simulink model "task_1"  (R2023b)
settings: Solver=FixedStepAuto  StartTime=0.0  StopTime=10  FixedStep=1e-3  RelTol=1e-3
values from neighbouring files (symbols this model uses):
  lambda = 4    [task_1.m]
  theta = 6    [task_1.m]
  x_init = 8    [task_1.m]
  x_m_init = 7    [task_1.m]
settings Model: Creator=nguye  LastModifiedBy=nguye

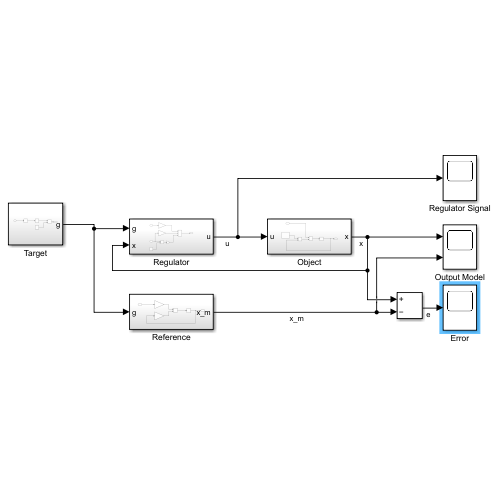
[thumbnail: Simulink's stored preview of the top-level diagram]
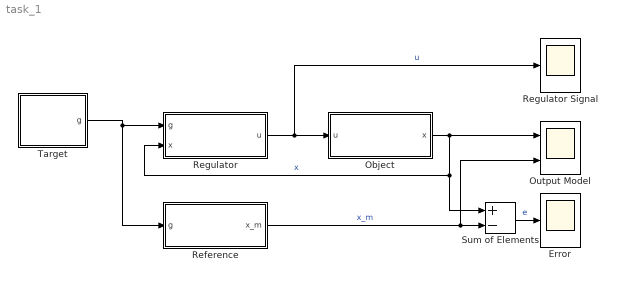
== system task_1 ==
  Error : Scope
  Object : Subsystem
  Output Model : Scope  NumInputPorts=2
  Reference : Subsystem
  Regulator : Subsystem
  Regulator Signal : Scope
  Sum of Elements : Sum  Inputs=+-
  Target : Subsystem
  wires:
  Target/1(g) -> Reference/1(g), Regulator/1(g)
  Regulator/1(u) -> Regulator Signal/1, Object/1(u)  "u"
  Object/1(x) -> Output Model/1, Sum of Elements/1, Regulator/2(x)  "x"
  Reference/1(x_m) -> Output Model/2, Sum of Elements/2  "x_m"
  Sum of Elements/1 -> Error/1  "e"

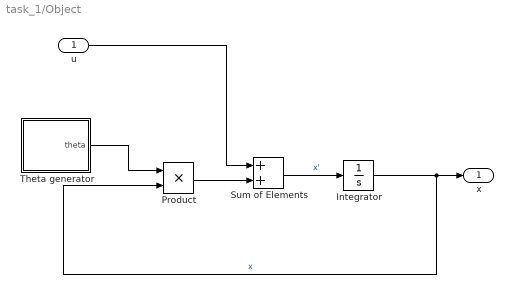
== system task_1/Object ==
  u : Inport
  Integrator : Integrator  InitialCondition=x_init
  Product : Product
  Sum of Elements : Sum
  Theta generator : Subsystem
  x : Outport
  wires:
  Integrator/1 -> Product/2, x/1  "x"
  Product/1 -> Sum of Elements/2
  Sum of Elements/1 -> Integrator/1  "x'"
  u/1 -> Sum of Elements/1
  Theta generator/1(theta) -> Product/1

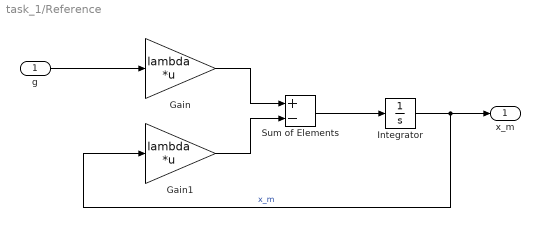
== system task_1/Reference ==
  g : Inport
  Gain : Gain  Gain=lambda  Multiplication=Matrix(K*u)
  Gain1 : Gain  Gain=lambda  Multiplication=Matrix(K*u)
  Integrator : Integrator  InitialCondition=x_m_init
  Sum of Elements : Sum  Inputs=+-
  x_m : Outport
  wires:
  Sum of Elements/1 -> Integrator/1
  Integrator/1 -> Gain1/1, x_m/1  "x_m"
  Gain/1 -> Sum of Elements/1
  g/1 -> Gain/1
  Gain1/1 -> Sum of Elements/2

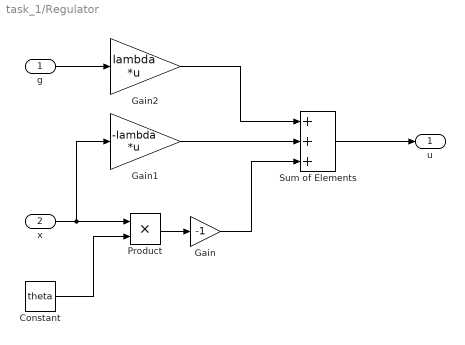
== system task_1/Regulator ==
  g : Inport
  x : Inport  Port=2
  Constant : Constant  Value=theta
  Gain : Gain  Gain=-1
  Gain1 : Gain  Gain=-lambda  Multiplication=Matrix(K*u)
  Gain2 : Gain  Gain=lambda  Multiplication=Matrix(K*u)
  Product : Product
  Sum of Elements : Sum  Inputs=+++
  u : Outport
  wires:
  x/1 -> Product/1, Gain1/1
  g/1 -> Gain2/1
  Sum of Elements/1 -> u/1
  Gain2/1 -> Sum of Elements/1
  Gain1/1 -> Sum of Elements/2
  Product/1 -> Gain/1
  Constant/1 -> Product/2
  Gain/1 -> Sum of Elements/3

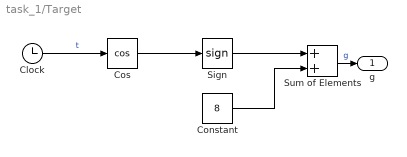
== system task_1/Target ==
  Clock : Clock
  Constant : Constant  Value=8
  Cos : Trigonometry  Operator=cos
  Sign : Signum
  Sum of Elements : Sum
  g : Outport
  wires:
  Clock/1 -> Cos/1  "t"
  Cos/1 -> Sign/1
  Sign/1 -> Sum of Elements/1
  Constant/1 -> Sum of Elements/2
  Sum of Elements/1 -> g/1  "g"

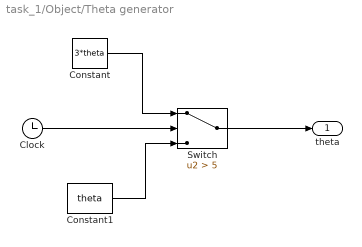
== system task_1/Object/Theta generator ==
  Clock : Clock
  Constant : Constant  Value=3*theta
  Constant1 : Constant  Value=theta
  Switch : Switch  Criteria=u2 > Threshold  Threshold=5  SaturateOnIntegerOverflow=off  InputSameDT=off
  theta : Outport
  wires:
  Clock/1 -> Switch/2
  Constant/1 -> Switch/1
  Constant1/1 -> Switch/3
  Switch/1 -> theta/1
